simulink model "massPID_variableGain"  (R2024a)
settings: Solver=FixedStepAuto  StartTime=0.0  StopTime=stopTime  FixedStep=1e-4  MaxStep=Tsample  RelTol=1e-8
values from neighbouring files (symbols this model uses):
  amp_d = 1    [runsim.m]
  Ap = [0, 1;0, 0]    [runsim.m]
  Bp = [0;1]    [runsim.m]
  Cp = eye(2)    [runsim.m]
  Dp = [0;0]    [runsim.m]
  high_gain = 2    [runsim.m]
  init_cond = [0;0]    [runsim.m]
  kd = 1e2    (= 100)    [runsim.m]
  ki = 5e6    (= 5000000)    [runsim.m]
  kp = 1e5    (= 100000)    [runsim.m]
undefined symbols (not defined in the file or in its folder): t_off
settings Model: Creator=chukh  LastModifiedBy=bengo
settings SolverCC: ZeroCrossAlgorithm=Adaptive  AlgebraicLoopSolver=TrustRegion
settings DebuggingCC: IgnoredZcDiagnostic=none  ArithmeticOperatorsInVariantConditions=warning
settings SFSimCC: CustomCodeUndefinedFunction=UseInterfaceOnly
settings RTWCC: GPUComputeCapability=3.5
settings CodeAppCC: StateflowObjectComments=on

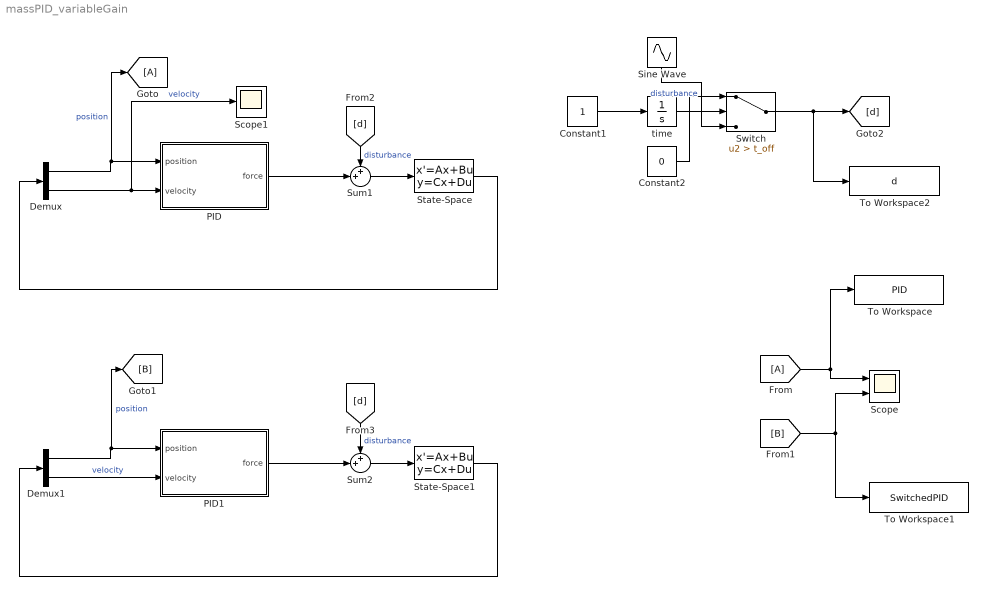
== system massPID_variableGain ==
  Constant1 : Constant
  Constant2 : Constant  Value=0
  Demux : Demux  Outputs=2
  Demux1 : Demux  Outputs=2
  From : From
  Goto : Goto
  PID : Subsystem
  PID1 : Subsystem
  Scope : Scope  NumInputPorts=2
  Scope1 : Scope
  Sine Wave : Sin  Amplitude=amp_d  Frequency=310  SampleTime=0
  State-Space : StateSpace  A=Ap  B=Bp  C=Cp  D=Dp  InitialCondition=init_cond
  State-Space1 : StateSpace  A=Ap  B=Bp  C=Cp  D=Dp  InitialCondition=init_cond
  Sum1 : Sum  Inputs=++|
  Sum2 : Sum  Inputs=++|
  Switch : Switch  Criteria=u2 > Threshold  Threshold=t_off  SaturateOnIntegerOverflow=off  InputSameDT=off
  To Workspace : ToWorkspace  VariableName=PID  SaveFormat=Timeseries  SampleTime=-1
  To Workspace1 : ToWorkspace  VariableName=SwitchedPID  SaveFormat=Timeseries  SampleTime=-1
  To Workspace2 : ToWorkspace  VariableName=d  SaveFormat=Timeseries  SampleTime=-1
  time : Integrator
  wires:
  State-Space/1 -> Demux/1
  Sum1/1 -> State-Space/1
  [d] -> Sum1/1  "disturbance"
  Demux/1 -> Goto/1, PID/1(position)  "position"
  Demux/2 -> Scope1/1, PID/2(velocity)  "velocity"
  PID/1(force) -> Sum1/2
  From/1 -> To Workspace/1, Scope/1
  [B] -> To Workspace1/1, Scope/2
  PID1/1(force) -> Sum2/2
  State-Space1/1 -> Demux1/1
  [d] -> Sum2/1  "disturbance"
  Demux1/2 -> PID1/2(velocity)  "velocity"
  Demux1/1 -> [B], PID1/1(position)  "position"
  Sum2/1 -> State-Space1/1
  Sine Wave/1 -> Switch/3  "disturbance"
  Switch/1 -> To Workspace2/1, [d]
  Constant1/1 -> time/1
  time/1 -> Switch/2
  Constant2/1 -> Switch/1

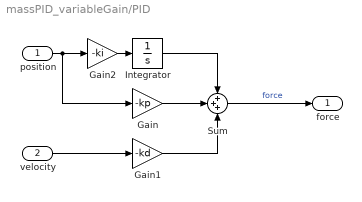
== system massPID_variableGain/PID ==
  position : Inport
  velocity : Inport  Port=2
  Gain : Gain  Gain=-kp
  Gain1 : Gain  Gain=-kd
  Gain2 : Gain  Gain=-ki
  Integrator : Integrator
  Sum : Sum  Inputs=+++
  force : Outport
  wires:
  velocity/1 -> Gain1/1
  Integrator/1 -> Sum/1
  Gain2/1 -> Integrator/1
  Gain/1 -> Sum/2
  Gain1/1 -> Sum/3
  position/1 -> Gain/1, Gain2/1
  Sum/1 -> force/1  "force"

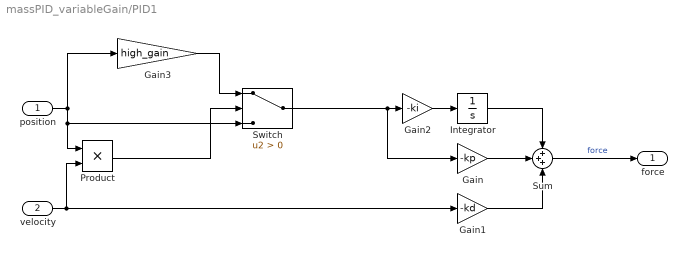
== system massPID_variableGain/PID1 ==
  position : Inport
  velocity : Inport  Port=2
  Gain : Gain  Gain=-kp
  Gain1 : Gain  Gain=-kd
  Gain2 : Gain  Gain=-ki
  Gain3 : Gain  Gain=high_gain
  Integrator : Integrator
  Product : Product
  Sum : Sum  Inputs=+++
  Switch : Switch  Criteria=u2 > Threshold  SaturateOnIntegerOverflow=off  InputSameDT=off
  force : Outport
  wires:
  velocity/1 -> Product/2, Gain1/1
  Integrator/1 -> Sum/1
  Gain2/1 -> Integrator/1
  Gain/1 -> Sum/2
  Gain1/1 -> Sum/3
  Switch/1 -> Gain/1, Gain2/1
  Sum/1 -> force/1  "force"
  position/1 -> Switch/3, Product/1, Gain3/1
  Product/1 -> Switch/2
  Gain3/1 -> Switch/1
